simulink model "Refined_Model_1"  (R2020b)
settings: Solver=ode8  StartTime=0.0  StopTime=250  FixedStep=dt  RelTol=1e-3
values from neighbouring files (symbols this model uses):
  CovDist = RoadProfile(:,4)    [ICE_Val.m]
  Cx = VehicleDefine(7,3)    [BEV_Basictest.m]    (also in GPS_val.m; ICEBEV_Script.m; ICEBEV_Script_VECTO.m; ICE_Script.m)
  DynRolRad = VehicleDefine(5,3)    [BEV_Basictest.m]    (also in GPS_val.m; ICEBEV_Script.m; ICEBEV_Script_VECTO.m; ICE_Script.m)
  EngineRpm = round(IntpTorCur(:,1))    [GPS_val.m]    (also in ICEBEV_Script.m; ICEBEV_Script_VECTO.m; ICE_Script.m; ICE_Script_SSVal.m)
  etaClutch = VehicleDefine(23,3)    [GPS_val.m]    (also in ICEBEV_Script.m; ICEBEV_Script_VECTO.m; ICE_Script.m; ICE_Script_SSVal.m)
  etaGRa = GBXDefine(:,3)    [GPS_val.m]    (also in ICEBEV_Script.m; ICEBEV_Script_VECTO.m; ICE_Script.m; ICE_Script_SSVal.m)
  FDR = VehicleDefine(20,3)    [BEV_Basictest.m]    (also in GPS_val.m = VehicleDefine(22,3); ICEBEV_Script.m = VehicleDefine(22,3); ICEBEV_Script_VECTO.m = VehicleDefine(22,3); ICE_Script.m = VehicleDefine(22,3))
  Fr = VehicleDefine(13,3)    [BEV_Basictest.m]    (also in GPS_val.m; ICEBEV_Script.m; ICEBEV_Script_VECTO.m; ICE_Script.m)
  g = VehicleDefine(14,3)    [BEV_Basictest.m]    (also in GPS_val.m; ICEBEV_Script.m; ICEBEV_Script_VECTO.m; ICE_Script.m)
  GNo = GBXDefine(:,1)    [GPS_val.m]    (also in ICEBEV_Script.m; ICEBEV_Script_VECTO.m; ICE_Script.m; ICE_Script_SSVal.m)
  GRa = GBXDefine(:,2)    [GPS_val.m]    (also in ICEBEV_Script.m; ICEBEV_Script_VECTO.m; ICE_Script.m; ICE_Script_SSVal.m)
  InitVel = VehicleDefine(21,3)    [BEV_Basictest.m]    (also in GPS_val.m = VehicleDefine(24,3); ICEBEV_Script.m = VehicleDefine(24,3); ICEBEV_Script_VECTO.m = VehicleDefine(24,3); ICE_Script.m = VehicleDefine(24,3))
  IntpSlope = round(IntpSlope,1)    [GPS_val.m]    (also in ICE_Script.m; ICE_Val.m = A)
  Jk = VehicleDefine(15,3)    [BEV_Basictest.m]    (also in GPS_val.m; ICEBEV_Script.m; ICEBEV_Script_VECTO.m; ICE_Script.m)
  Jm = VehicleDefine(16,3)    [GPS_val.m]    (also in ICEBEV_Script.m; ICEBEV_Script_VECTO.m; ICE_Script.m; ICE_Script_SSVal.m)
  MaxSpeedProfile = FMSP    [GPS_val.m]    (also in ICE_Script.m; ICE_Val.m = repelem(SegSPLatinmps,SegLeninm))
  MaxTorValThrot = max(ThrotTableVal,[],2)    [GPS_val.m]    (also in ICEBEV_Script.m; ICEBEV_Script_VECTO.m; ICE_Script.m; ICE_Script_SSVal.m)
  Me = VehicleDefine(10,3)    [BEV_Basictest.m]    (also in GPS_val.m; ICEBEV_Script.m; ICEBEV_Script_VECTO.m; ICE_Script.m)
  MotoringTor = IntpTorCur(:,3)    [GPS_val.m]    (also in ICEBEV_Script.m; ICEBEV_Script_VECTO.m; ICE_Script.m; ICE_Script_SSVal.m)
  Mt = VehicleDefine(12,3)    [BEV_Basictest.m]    (also in GPS_val.m; ICEBEV_Script.m; ICEBEV_Script_VECTO.m; ICE_Script.m)
  Mtot = Mv+Me+Mt    [BEV_Basictest.m]    (also in GPS_val.m; ICEBEV_Script.m; ICEBEV_Script_VECTO.m; ICE_Script.m)
  Mv = VehicleDefine(9,3)    [BEV_Basictest.m]    (also in GPS_val.m; ICEBEV_Script.m; ICEBEV_Script_VECTO.m; ICE_Script.m)
  NoSteps = round(Dist(end))    [GPS_val.m]    (also in ICE_Script.m; ICE_Val.m = 3002)
  NoWhlFA = VehicleDefine(2,3)    [BEV_Basictest.m]    (also in GPS_val.m; ICE_Script.m; ICE_Val.m; ICE_Val_new.m)
  NoWhlRA = VehicleDefine(4,3)    [BEV_Basictest.m]    (also in GPS_val.m; ICE_Script.m; ICE_Val.m; ICE_Val_new.m)
  rho = VehicleDefine(6,3)    [BEV_Basictest.m]    (also in GPS_val.m; ICEBEV_Script.m; ICEBEV_Script_VECTO.m; ICE_Script.m)
  RpmBrkPnt = ThrottleMap(1,:)    [GPS_val.m]    (also in ICEBEV_Script.m; ICEBEV_Script_VECTO.m; ICE_Script.m; ICE_Script_SSVal.m)
  SegNo = RoadProfile(:,1)    [ICE_Val.m]
  SegSPLatinmps = (sqrt(aMaxLat*g*CurRadinm))    [GPS_val.m]    (also in ICE_Script.m; ICE_Val.m)
  Sx = VehicleDefine(8,3)    [BEV_Basictest.m]    (also in GPS_val.m; ICEBEV_Script.m; ICEBEV_Script_VECTO.m; ICE_Script.m)
  ThrotPos = ThrotPos'    [GPS_val.m]    (also in ICEBEV_Script.m; ICEBEV_Script_VECTO.m; ICE_Script.m; ICE_Script_SSVal.m)
  ThrotTableVal = ThrottleMap(2:end,2:end)    [GPS_val.m]    (also in ICEBEV_Script.m; ICEBEV_Script_VECTO.m; ICE_Script.m; ICE_Script_SSVal.m)
undefined symbols (not defined in the file or in its folder): AccLim, G1Inprpm, GearNo, GInprpm, GInpTor, GTorLoss, MaxSpinG, MaxWhlTorinG
libraries: simulink x2
settings Model: Creator=Kshitij  LastModifiedBy=Kshitij
settings SolverCC: AutoInsertRateTranBlk=on
settings DataIOCC: SaveFinalState=on  SaveState=on  InspectSignalLogs=on
settings DebuggingCC: AlgebraicLoopMsg=none
settings SFSimCC: SimTargetLang=C++  GPUAcceleration=on  SimDLTargetLibrary=cudnn

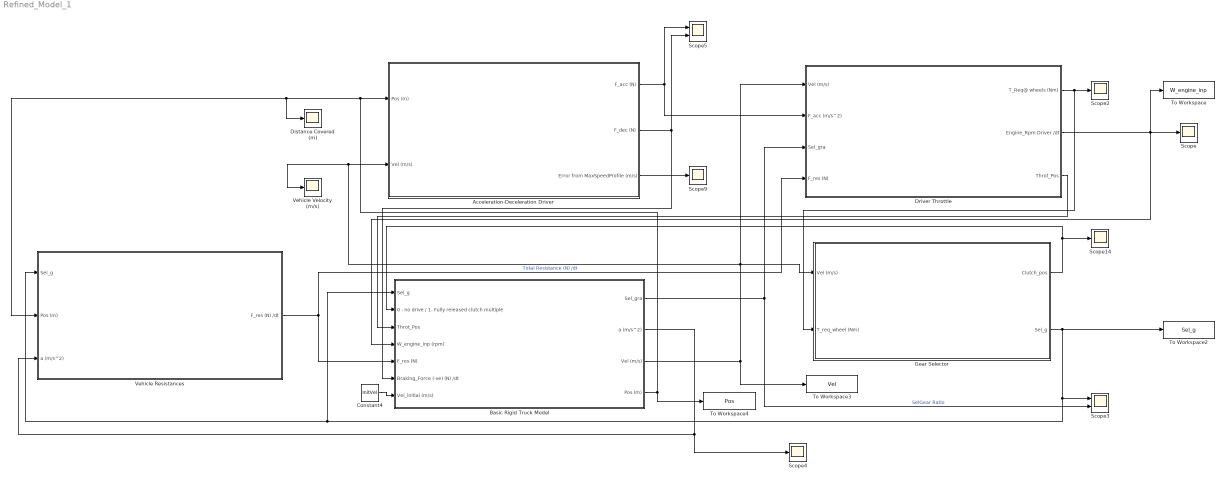
== system Refined_Model_1 ==
  Acceleration-Deceleration Driver : Subsystem
  Basic Rigid Truck Model : Subsystem
  Constant4 : Constant  Value=InitVel
  Distance Covered (m) : Scope
  Driver Throttle : Subsystem
  Gear Selector : Subsystem
  Scope{,2,4,9,14} (5 alike) : Scope
  Scope3 : Scope  NumInputPorts=2
  Scope5 : Scope  NumInputPorts=2
  To Workspace : ToWorkspace  VariableName=W_engine_inp  SaveFormat=Timeseries  SampleTime=-1
  To Workspace2 : ToWorkspace  VariableName=Sel_g  SaveFormat=Timeseries  SampleTime=-1
  To Workspace3 : ToWorkspace  VariableName=Vel  SaveFormat=Timeseries  SampleTime=-1
  To Workspace4 : ToWorkspace  VariableName=Pos  SaveFormat=Timeseries  SampleTime=-1
  Vehicle Resistances : Subsystem
  Vehicle Velocity (m/s) : Scope
  wires:
  Basic Rigid Truck Model/4(Pos (m)) -> Acceleration-Deceleration Driver/1(Pos (m)), Distance Covered (m)/1, Vehicle Resistances/2(Pos (m)), To Workspace4/1
  Vehicle Resistances/1(F_res (N) /dt) -> Basic Rigid Truck Model/5(F_res (N)), Driver Throttle/4(F_res (N))  "Total Resistance (N) /dt"
  Basic Rigid Truck Model/2(a (m/s^2)) -> Scope4/1, Vehicle Resistances/3(a (m/s^2))
  Gear Selector/1(Clutch_pos) -> Basic Rigid Truck Model/2(0 - no drive / 1- Fully released clutch multiple), Scope14/1
  Gear Selector/2(Sel_g) -> To Workspace2/1, Basic Rigid Truck Model/1(Sel_g), Vehicle Resistances/1(Sel_g), Scope3/1
  Acceleration-Deceleration Driver/3(Error from MaxSpeedProfile (m/s)) -> Scope9/1
  Acceleration-Deceleration Driver/2(F_dec (N)) -> Basic Rigid Truck Model/6(Braking_Force (-ve) (N) /dt), Scope5/2
  Basic Rigid Truck Model/1(Sel_gra) -> Driver Throttle/3(Sel_gra), Scope3/2  "SelGear Ratio"
  Acceleration-Deceleration Driver/1(F_acc (N)) -> Scope5/1, Driver Throttle/2(F_acc (m/s^2))
  Driver Throttle/2(Engine_Rpm Driver /dt) -> To Workspace/1, Scope/1, Basic Rigid Truck Model/4(W_engine_inp (rpm))
  Driver Throttle/1(T_Req@ wheels (Nm)) -> Gear Selector/2(T_req_wheel (Nm)), Scope2/1
  Constant4/1 -> Basic Rigid Truck Model/7(Vel_initial (m/s))
  Basic Rigid Truck Model/3(Vel (m/s)) -> Driver Throttle/1(Vel (m/s)), Vehicle Velocity (m/s)/1, Acceleration-Deceleration Driver/2(Vel (m/s)), Gear Selector/1(Vel (m/s)), To Workspace3/1
  Driver Throttle/3(Throt_Pos) -> Basic Rigid Truck Model/3(Throt_Pos)

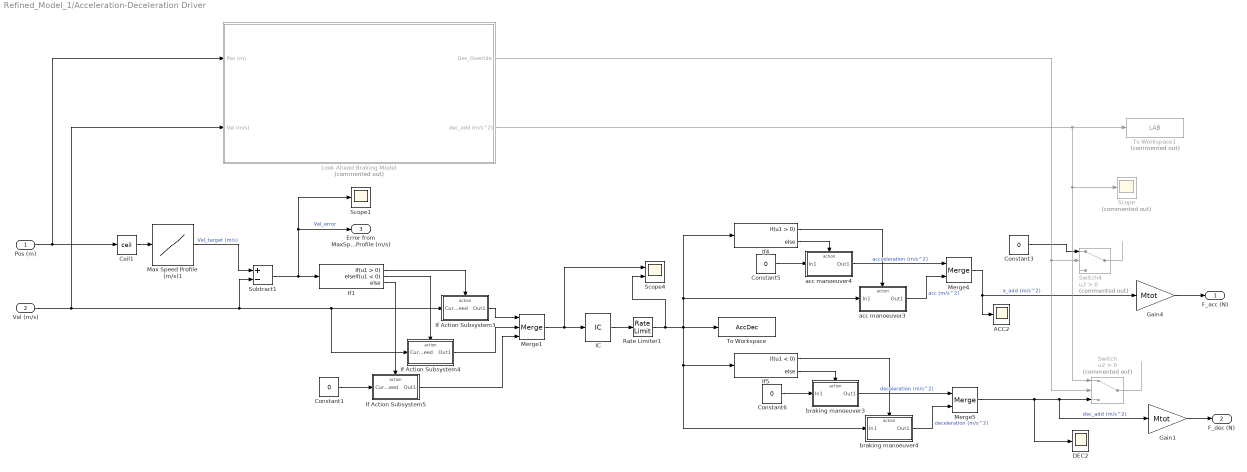
== system Refined_Model_1/Acceleration-Deceleration Driver ==
  Pos (m) : Inport
  Vel (m/s) : Inport  Port=2
  ACC2 : Scope
  Ceil1 : Rounding  Operator=ceil
  Constant{1,3,5..6} (4 alike) : Constant  Value=0
  DEC2 : Scope
  Gain1 : Gain  Gain=Mtot
  Gain4 : Gain  Gain=Mtot
  IC : InitialCondition  Value=0
  If Action Subsystem3 : Subsystem  TreatAsAtomicUnit=on
  If Action Subsystem4 : Subsystem  TreatAsAtomicUnit=on
  If Action Subsystem5 : Subsystem  TreatAsAtomicUnit=on
  If1 : If  ElseIfExpressions=u1 < 0
  If4 : If
  If5 : If  IfExpression=u1 < 0
  Look Ahead Braking Model : Subsystem  Commented=on
  Max Speed Profile (m/s)1 : Lookup_n-D  NumberOfTableDimensions=1  BreakpointsForDimension1=[1:length(MaxSpeedProfile)]  BreakpointsForDimension2=G1Inprpm  Table=MaxSpeedProfile  InterpMethod=Linear Lagrange  InternalRulePriority=Speed  RndMeth=Simplest  InputSameDT=on
  Merge1 : Merge  Inputs=3
  Merge4 : Merge
  Merge5 : Merge
  Rate Limiter1 : RateLimiter  RisingSlewLimit=0.5  SampleTimeMode=inherited
  Scope : Scope  Commented=on
  Scope1 : Scope
  Scope4 : Scope  NumInputPorts=2
  Subtract1 : Sum  Inputs=+-
  Switch : Switch  Commented=on  Criteria=u2 > Threshold
  Switch4 : Switch  Commented=on  Criteria=u2 > Threshold
  To Workspace : ToWorkspace  VariableName=AccDec  SaveFormat=Timeseries  SampleTime=-1
  To Workspace1 : ToWorkspace  Commented=on  VariableName=LAB  SaveFormat=Timeseries  SampleTime=-1
  acc manoeuver3 : Subsystem  TreatAsAtomicUnit=on
  acc manoeuver4 : Subsystem  TreatAsAtomicUnit=on
  braking manoeuver3 : Subsystem  TreatAsAtomicUnit=on
  braking manoeuver4 : Subsystem  TreatAsAtomicUnit=on
  F_acc (N) : Outport
  F_dec (N) : Outport  Port=2
  Error from MaxSpeedProfile (m/s) : Outport  Port=3
  wires:
  acc manoeuver4/1(Out1) -> Merge4/1  "accceleration (m/s^2)"
  If Action Subsystem3/1(Out1) -> Merge1/1
  If Action Subsystem5/1(Out1) -> Merge1/3
  Ceil1/1 -> Max Speed Profile (m/s)1/1
  If5/2 -> braking manoeuver3/Action
  Pos (m)/1 -> Look Ahead Braking Model/1(Pos (m)), Ceil1/1
  If1/1 -> If Action Subsystem3/Action
  If5/1 -> braking manoeuver4/Action
  Constant5/1 -> acc manoeuver4/1(In1)
  braking manoeuver3/1(Out1) -> Merge5/1  "deceleration (m/s^2)"
  braking manoeuver4/1(Out1) -> Merge5/2  "deceleration (m/s^2)"
  Constant6/1 -> braking manoeuver3/1(In1)
  Merge5/1 -> Gain1/1, Switch/3, DEC2/1  "dec_add (m/s^2)"
  If Action Subsystem4/1(Out1) -> Merge1/2
  acc manoeuver3/1(Out1) -> Merge4/2  "acc (m/s^2)"
  Merge4/1 -> ACC2/1, Gain4/1  "a_add (m/s^2)"
  If1/2 -> If Action Subsystem4/Action
  Subtract1/1 -> Error from MaxSpeedProfile (m/s)/1, Scope1/1, If1/1  "Vel_error"
  Rate Limiter1/1 -> Scope4/2, If4/1, acc manoeuver3/1(In1), If5/1, braking manoeuver4/1(In1), To Workspace/1
  If4/2 -> acc manoeuver4/Action
  If4/1 -> acc manoeuver3/Action
  If1/3 -> If Action Subsystem5/Action
  Merge1/1 -> IC/1, Scope4/1
  Max Speed Profile (m/s)1/1 -> Subtract1/1  "Vel_target (m/s)"
  Vel (m/s)/1 -> Look Ahead Braking Model/2(Vel (m/s)), If Action Subsystem4/1(Current Speed), If Action Subsystem3/1(Current Speed), Subtract1/2
  Constant1/1 -> If Action Subsystem5/1(Current Speed)
  IC/1 -> Rate Limiter1/1
  Constant3/1 -> Switch4/1
  Look Ahead Braking Model/1(Dec_Override) -> Switch/2, Switch4/2
  Look Ahead Braking Model/2(dec_add (m/s^2)) -> To Workspace1/1, Scope/1, Switch/1
  Gain4/1 -> F_acc (N)/1
  Switch4/1 -> ?
  Gain1/1 -> F_dec (N)/1
  Switch/1 -> ?

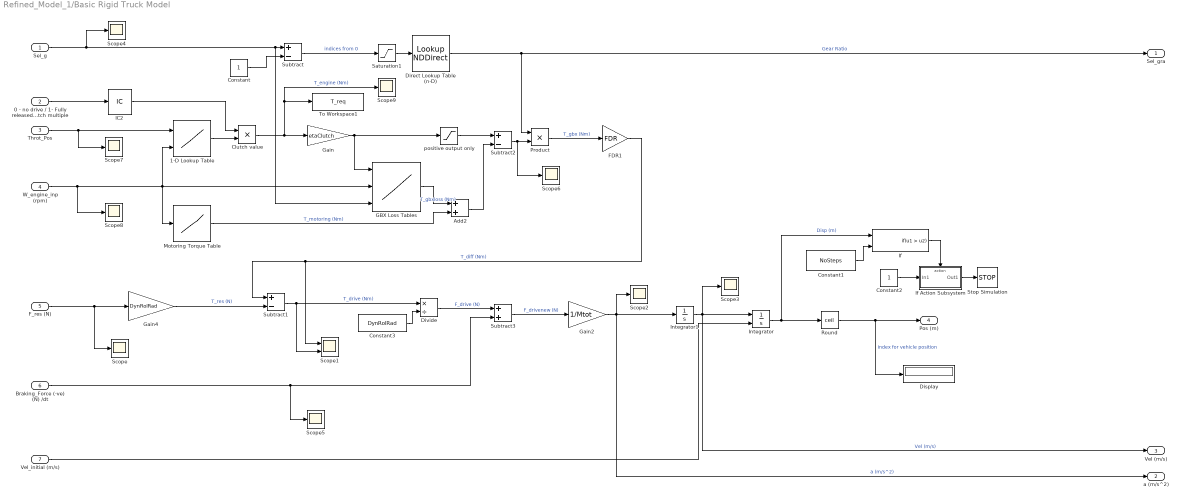
== system Refined_Model_1/Basic Rigid Truck Model ==
  Sel_g : Inport
  0 - no drive / 1- Fully released clutch multiple : Inport  Port=2
  Throt_Pos : Inport  Port=3
  W_engine_inp (rpm) : Inport  Port=4
  F_res (N) : Inport  Port=5
  Braking_Force (-ve) (N) /dt : Inport  Port=6
  Vel_initial (m/s) : Inport  Port=7
  1-D Lookup Table : Lookup_n-D  BreakpointsForDimension1=ThrotPos  BreakpointsForDimension2=RpmBrkPnt  Table=ThrotTableVal  InternalRulePriority=Speed  RndMeth=Simplest  InputSameDT=on
      settings: InputPortMap=u0,u1
  Add2 : Sum
  Clutch value : Product
  Constant : Constant
  Constant1 : Constant  Value=NoSteps
  Constant2 : Constant
  Constant3 : Constant  Value=DynRolRad
  Direct Lookup Table (n-D) : LookupNDDirect  NumberOfTableDimensions=1  Table=GRa
  Display : Display
  Divide : Product  Inputs=*/
  FDR1 : Gain  Gain=FDR
  GBX Loss Tables : Lookup_n-D  NumberOfTableDimensions=3  BreakpointsForDimension1=GInpTor  BreakpointsForDimension2=GInprpm  BreakpointsForDimension3=GearNo  Table=GTorLoss  InterpMethod=Linear Lagrange  InternalRulePriority=Speed  RndMeth=Simplest  InputSameDT=on
      settings: InputPortMap=u0,u1,u2
  Gain : Gain  Gain=etaClutch
  Gain2 : Gain  Gain=1/Mtot
  Gain4 : Gain  Gain=DynRolRad
  IC2 : InitialCondition
  If : If  NumInputs=2  IfExpression=u1 > u2  ShowElse=off
  If Action Subsystem : Subsystem  TreatAsAtomicUnit=on
  Integrator : Integrator  InitialConditionSource=external  ContinuousStateAttributes='velocity'
  Integrator1 : Integrator  ContinuousStateAttributes='acceleration'
  Motoring Torque Table : Lookup_n-D  NumberOfTableDimensions=1  BreakpointsForDimension1=EngineRpm  BreakpointsForDimension2=G1Inprpm  Table=MotoringTor  InterpMethod=Linear Lagrange  InternalRulePriority=Speed  RndMeth=Simplest  InputSameDT=on
  Product : Product
  Round : Rounding  Operator=ceil
  Saturation1 : Saturate  UpperLimit=inf  LowerLimit=0
  Scope{,2..9} (9 alike) : Scope
  Scope1 : Scope  NumInputPorts=2
  Stop Simulation : Stop
  Subtract : Sum  Inputs=+-
  Subtract1 : Sum  Inputs=+-
  Subtract2 : Sum  Inputs=+-
  Subtract3 : Sum
  To Workspace1 : ToWorkspace  VariableName=T_req  SaveFormat=Timeseries  SampleTime=-1
  positive output only : Saturate  UpperLimit=max(MaxTorValThrot)  LowerLimit=0
  Sel_gra : Outport
  a (m/s^2) : Outport  Port=2
  Vel (m/s) : Outport  Port=3
  Pos (m) : Outport  Port=4
  wires:
  GBX Loss Tables/1 -> Add2/1  "T_gbxloss (Nm)"
  Motoring Torque Table/1 -> Add2/2  "T_motoring (Nm)"
  FDR1/1 -> Subtract1/1, Scope1/1  "T_diff (Nm)"
  Direct Lookup Table (n-D)/1 -> Sel_gra/1, Product/1  "Gear Ratio"
  Clutch value/1 -> To Workspace1/1, Scope9/1, Gain/1  "T_engine (Nm)"
  Gain4/1 -> Subtract1/2  "T_res (N)"
  Subtract1/1 -> Divide/1, Scope1/2  "T_drive (Nm)"
  Add2/1 -> Subtract2/2
  Subtract2/1 -> Scope6/1, Product/2
  0 - no drive / 1- Fully released clutch multiple/1 -> IC2/1
  F_res (N)/1 -> Scope/1, Gain4/1
  Divide/1 -> Subtract3/1  "F_drive (N)"
  positive output only/1 -> Subtract2/1
  Sel_g/1 -> Scope4/1, Subtract/1, GBX Loss Tables/3
  Subtract/1 -> Saturation1/1  "indices from 0"
  Constant/1 -> Subtract/2
  Subtract3/1 -> Gain2/1  "F_drivenew (N)"
  Gain2/1 -> Integrator1/1, Scope2/1, a (m/s^2)/1  "a (m/s^2)"
  1-D Lookup Table/1 -> Clutch value/2
  Product/1 -> FDR1/1  "T_gbx (Nm)"
  Gain/1 -> positive output only/1, GBX Loss Tables/1
  W_engine_inp (rpm)/1 -> Scope8/1, Motoring Torque Table/1, GBX Loss Tables/2, 1-D Lookup Table/2
  IC2/1 -> Clutch value/1
  If/1 -> If Action Subsystem/Action
  Integrator1/1 -> Integrator/1, Scope3/1, Vel (m/s)/1  "Vel (m/s)"
  Constant1/1 -> If/2
  If Action Subsystem/1(Out1) -> Stop Simulation/1
  Round/1 -> Pos (m)/1, Display/1  "Index for vehicle position"
  Constant2/1 -> If Action Subsystem/1(In1)
  Integrator/1 -> Round/1, If/1  "Disp (m)"
  Constant3/1 -> Divide/2
  Vel_initial (m/s)/1 -> Integrator/2
  Saturation1/1 -> Direct Lookup Table (n-D)/1
  Throt_Pos/1 -> Scope7/1, 1-D Lookup Table/1
  Braking_Force (-ve) (N) /dt/1 -> Scope5/1, Subtract3/2

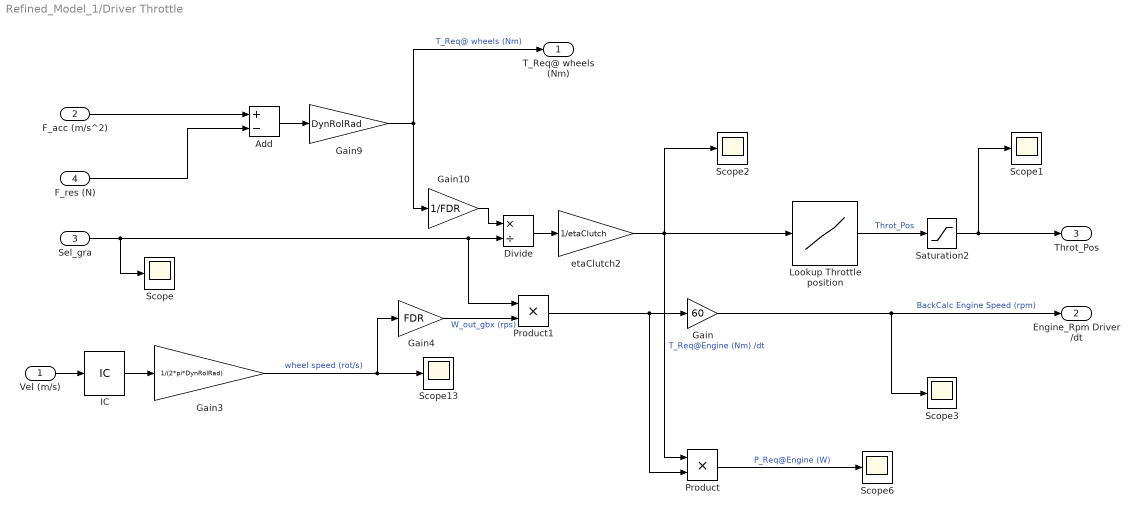
== system Refined_Model_1/Driver Throttle ==
  Vel (m/s) : Inport
  F_acc (m/s^2) : Inport  Port=2
  Sel_gra : Inport  Port=3
  F_res (N) : Inport  Port=4
  Add : Sum  Inputs=+-
  Divide : Product  Inputs=*/
  Gain : Gain  Gain=60
  Gain10 : Gain  Gain=1/FDR
  Gain3 : Gain  Gain=1/(2*pi*DynRolRad)
  Gain4 : Gain  Gain=FDR
  Gain9 : Gain  Gain=DynRolRad
  IC : InitialCondition  Value=0.1
  Lookup Throttle position : Lookup_n-D  NumberOfTableDimensions=1  BreakpointsForDimension1=MaxTorValThrot  Table=ThrotPos  InternalRulePriority=Speed  RndMeth=Simplest  InputSameDT=on
  Product : Product
  Product1 : Product
  Saturation2 : Saturate  UpperLimit=1  LowerLimit=0
  Scope{,1..3,6,13} (6 alike) : Scope
  etaClutch2 : Gain  Gain=1/etaClutch
  T_Req@ wheels (Nm) : Outport
  Engine_Rpm Driver /dt : Outport  Port=2
  Throt_Pos : Outport  Port=3
  wires:
  etaClutch2/1 -> Scope2/1, Lookup Throttle position/1, Product/1  "T_Req@Engine (Nm) /dt"
  Add/1 -> Gain9/1
  Gain4/1 -> Product1/2  "W_out_gbx (rps)"
  Product/1 -> Scope6/1  "P_Req@Engine (W)"
  Gain9/1 -> Gain10/1, T_Req@ wheels (Nm)/1  "T_Req@ wheels (Nm)"
  Gain3/1 -> Scope13/1, Gain4/1  "wheel speed (rot/s)"
  Gain10/1 -> Divide/1
  Sel_gra/1 -> Scope/1, Divide/2, Product1/1
  F_acc (m/s^2)/1 -> Add/1
  Vel (m/s)/1 -> IC/1
  Divide/1 -> etaClutch2/1
  F_res (N)/1 -> Add/2
  Product1/1 -> Gain/1, Product/2
  Lookup Throttle position/1 -> Saturation2/1  "Throt_Pos"
  Saturation2/1 -> Scope1/1, Throt_Pos/1
  IC/1 -> Gain3/1
  Gain/1 -> Engine_Rpm Driver /dt/1, Scope3/1  "BackCalc Engine Speed (rpm)"

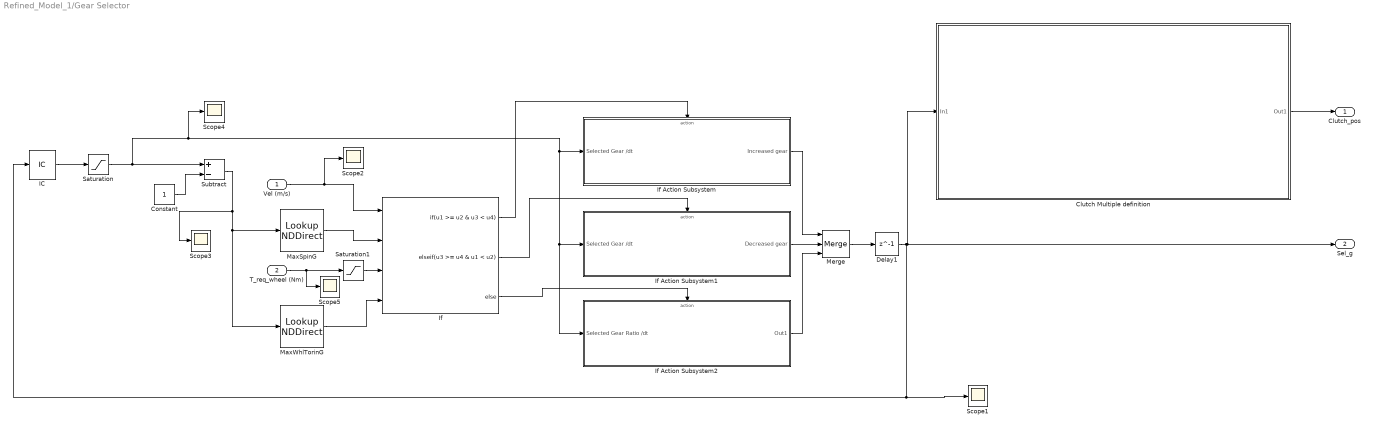
== system Refined_Model_1/Gear Selector ==
  Vel (m/s) : Inport
  T_req_wheel (Nm) : Inport  Port=2
  Clutch Multiple definition : Subsystem
  Constant : Constant
  Delay1 : Delay  DelayLength=1
  IC : InitialCondition
  If : If  NumInputs=4  IfExpression=u1 >= u2 & u3 < u4  ElseIfExpressions=u3 >= u4 & u1 < u2
  If Action Subsystem : Subsystem  TreatAsAtomicUnit=on
  If Action Subsystem1 : Subsystem  TreatAsAtomicUnit=on
  If Action Subsystem2 : Subsystem  TreatAsAtomicUnit=on
  MaxSpinG : LookupNDDirect  NumberOfTableDimensions=1  Table=MaxSpinG
  MaxWhlTorinG : LookupNDDirect  NumberOfTableDimensions=1  Table=MaxWhlTorinG
  Merge : Merge  Inputs=3
  Saturation : Saturate  UpperLimit=max(GNo)  LowerLimit=0
  Saturation1 : Saturate  UpperLimit=inf  LowerLimit=0
  Scope{1..5} (5 alike) : Scope
  Subtract : Sum  Inputs=+-
  Clutch_pos : Outport
  Sel_g : Outport  Port=2
  wires:
  If/1 -> If Action Subsystem/Action
  MaxWhlTorinG/1 -> If/4
  Vel (m/s)/1 -> Scope2/1, If/1
  MaxSpinG/1 -> If/2
  If/2 -> If Action Subsystem1/Action
  If Action Subsystem/1(Increased gear) -> Merge/1
  If Action Subsystem1/1(Decreased gear) -> Merge/2
  Constant/1 -> Subtract/2
  Subtract/1 -> Scope3/1, MaxSpinG/1, MaxWhlTorinG/1
  If/3 -> If Action Subsystem2/Action
  If Action Subsystem2/1(Out1) -> Merge/3
  Delay1/1 -> Clutch Multiple definition/1(In1), Sel_g/1, IC/1, Scope1/1
  Saturation/1 -> Subtract/1, If Action Subsystem2/1(Selected Gear Ratio /dt), If Action Subsystem1/1(Selected Gear /dt), If Action Subsystem/1(Selected Gear /dt), Scope4/1
  T_req_wheel (Nm)/1 -> Scope5/1, Saturation1/1
  Clutch Multiple definition/1(Out1) -> Clutch_pos/1
  Saturation1/1 -> If/3
  Merge/1 -> Delay1/1
  IC/1 -> Saturation/1

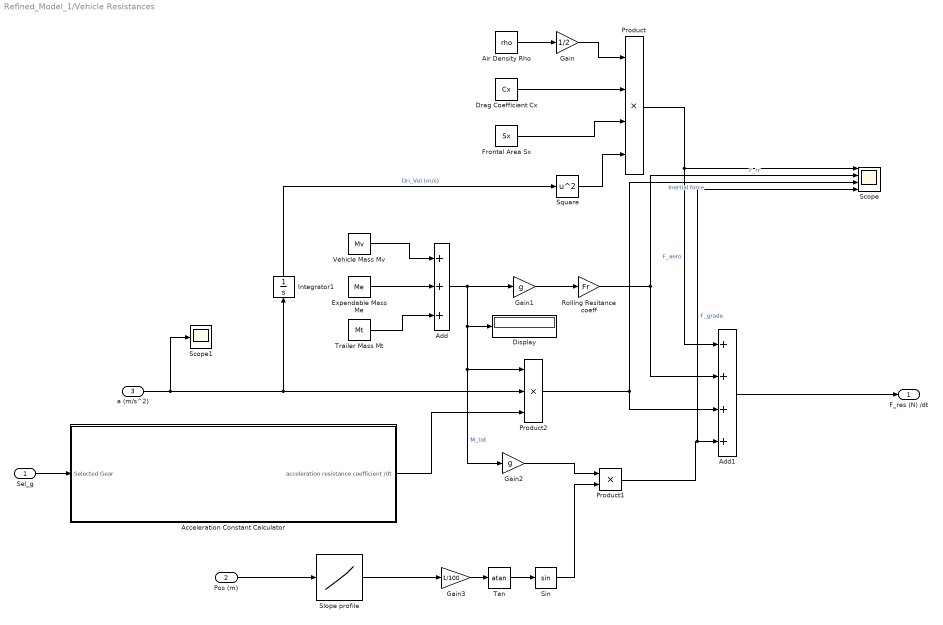
== system Refined_Model_1/Vehicle Resistances ==
  Sel_g : Inport
  Pos (m) : Inport  Port=2
  a (m/s^2) : Inport  Port=3
  Acceleration Constant Calculator : Subsystem
  Add : Sum  Inputs=+++
  Add1 : Sum  Inputs=++++
  Air Density Rho : Constant  Value=rho
  Display : Display
  Drag Coefficient Cx : Constant  Value=Cx
  Expendable Mass Me : Constant  Value=Me
  Frontal Area Sx : Constant  Value=Sx
  Gain : Gain  Gain=1/2
  Gain1 : Gain  Gain=g
  Gain2 : Gain  Gain=g
  Gain3 : Gain  Gain=1/100
  Integrator1 : Integrator
  Product : Product  Inputs=4
  Product1 : Product
  Product2 : Product  Inputs=3
  Rolling Resitance coeff : Gain  Gain=Fr
  Scope : Scope  NumInputPorts=4
  Scope1 : Scope
  Sin : Trigonometry
  Slope profile : Lookup_n-D  NumberOfTableDimensions=1  BreakpointsForDimension1=1: length(IntpSlope)  Table=IntpSlope  InternalRulePriority=Speed  RndMeth=Simplest  InputSameDT=on
  Square : Math  Operator=square  SaturateOnIntegerOverflow=on
  Tan : Trigonometry  Operator=atan
  Trailer Mass Mt : Constant  Value=Mt
  Vehicle Mass Mv : Constant  Value=Mv
  F_res (N) /dt : Outport
  wires:
  Expendable Mass Me/1 -> Add/2
  Add/1 -> Display/1, Gain2/1, Product2/1, Gain1/1  "M_tot"
  Gain/1 -> Product/1
  Sin/1 -> Product1/2
  Tan/1 -> Sin/1
  Product1/1 -> Scope/4, Add1/4  "F_grade"
  Air Density Rho/1 -> Gain/1
  Drag Coefficient Cx/1 -> Product/2
  Integrator1/1 -> Square/1  "Dri_Vel (m/s)"
  Pos (m)/1 -> Slope profile/1
  Gain2/1 -> Product1/1
  Trailer Mass Mt/1 -> Add/3
  Rolling Resitance coeff/1 -> Scope/2, Add1/2  "F_rr"
  Square/1 -> Product/4
  Gain1/1 -> Rolling Resitance coeff/1
  Vehicle Mass Mv/1 -> Add/1
  Product/1 -> Scope/1, Add1/1  "F_aero"
  Gain3/1 -> Tan/1
  Frontal Area Sx/1 -> Product/3
  Product2/1 -> Scope/3, Add1/3  "Inertial force"
  Acceleration Constant Calculator/1(acceleration resistance coefficient /dt) -> Product2/3
  Sel_g/1 -> Acceleration Constant Calculator/1(Selected Gear)
  Add1/1 -> F_res (N) /dt/1
  a (m/s^2)/1 -> Scope1/1, Product2/2, Integrator1/1
  Slope profile/1 -> Gain3/1

== system Refined_Model_1/Acceleration-Deceleration Driver/If Action Subsystem3 ==
  Current Speed : Inport
  Action Port : ActionPort  ActionPortLabel=if(u1 > 0)
  Acceleration : Lookup_n-D  NumberOfTableDimensions=1  BreakpointsForDimension1=AccLim(:,1)  Table=AccLim(:,2)  InternalRulePriority=Speed  RndMeth=Simplest  InputSameDT=on
  Out1 : Outport
  wires:
  Current Speed/1 -> Acceleration/1
  Acceleration/1 -> Out1/1  "Acceleration in m/s^2"

== system Refined_Model_1/Acceleration-Deceleration Driver/If Action Subsystem4 ==
  Current Speed : Inport
  Action Port : ActionPort  ActionPortLabel=elseif(u1 < 0)
  Deceleration : Lookup_n-D  NumberOfTableDimensions=1  BreakpointsForDimension1=AccLim(:,1)  Table=AccLim(:,3)  InternalRulePriority=Speed  RndMeth=Simplest  InputSameDT=on
  Out1 : Outport
  wires:
  Deceleration/1 -> Out1/1  "Acceleration in m/s^2"
  Current Speed/1 -> Deceleration/1

== system Refined_Model_1/Acceleration-Deceleration Driver/If Action Subsystem5 ==
  Current Speed : Inport
  Action Port : ActionPort  ActionPortLabel=else
  Out1 : Outport
  wires:
  Current Speed/1 -> Out1/1  "Acceleration in m/s^2"

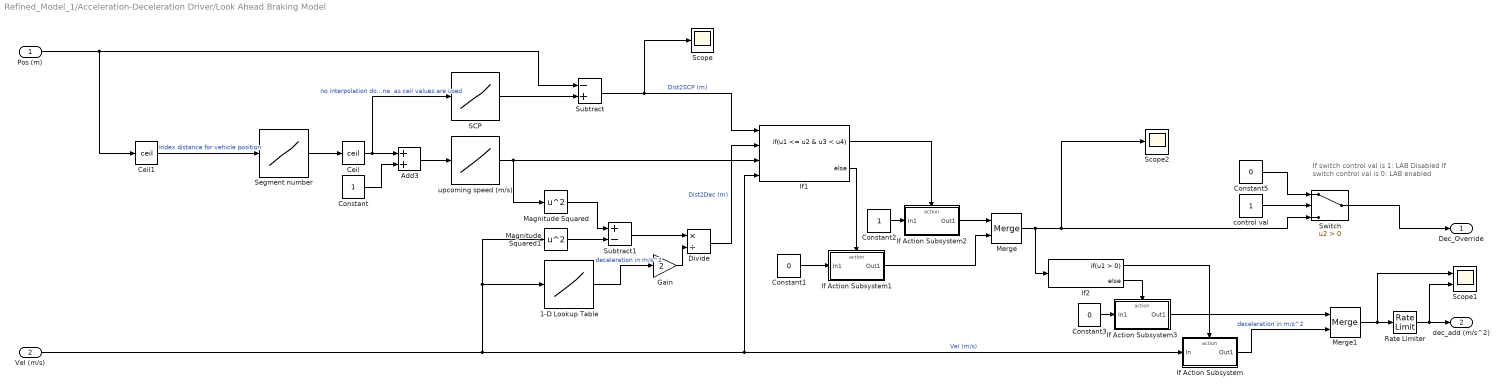
== system Refined_Model_1/Acceleration-Deceleration Driver/Look Ahead Braking Model ==
  note: If switch control val is 1: LAB Disabled
      | If switch control val is 0: LAB enabled
  Pos (m) : Inport
  Vel (m/s) : Inport  Port=2
  1-D Lookup Table : Lookup_n-D  NumberOfTableDimensions=1  BreakpointsForDimension1=AccLim(:,1)  Table=AccLim(:,3)  InternalRulePriority=Speed  RndMeth=Simplest  InputSameDT=on
  Add3 : Sum
  Ceil : Rounding  Operator=ceil
  Ceil1 : Rounding  Operator=ceil
  Constant : Constant
  Constant1 : Constant  Value=0
  Constant2 : Constant
  Constant3 : Constant  Value=0
  Constant5 : Constant  Value=0
  Divide : Product  Inputs=*/
  Gain : Gain  Gain=2
  If Action Subsystem : Subsystem  TreatAsAtomicUnit=on
  If Action Subsystem1 : Subsystem  TreatAsAtomicUnit=on
  If Action Subsystem2 : Subsystem  TreatAsAtomicUnit=on
  If Action Subsystem3 : Subsystem  TreatAsAtomicUnit=on
  If1 : If  NumInputs=4  IfExpression=u1 <= u2 & u3 < u4
  If2 : If
  Magnitude Squared : Math  Operator=square  SaturateOnIntegerOverflow=on
  Magnitude Squared1 : Math  Operator=square  SaturateOnIntegerOverflow=on
  Merge : Merge
  Merge1 : Merge
  Rate Limiter : RateLimiter  SampleTimeMode=inherited
  SCP : Lookup_n-D  NumberOfTableDimensions=1  BreakpointsForDimension1=SegNo  BreakpointsForDimension2=G1Inprpm  Table=CovDist  InterpMethod=Linear Lagrange  InternalRulePriority=Speed  RndMeth=Simplest  InputSameDT=on
  Scope : Scope
  Scope1 : Scope  NumInputPorts=2
  Scope2 : Scope
  Segment number : Lookup_n-D  NumberOfTableDimensions=1  BreakpointsForDimension1=CovDist  BreakpointsForDimension2=G1Inprpm  Table=SegNo  InterpMethod=Linear Lagrange  InternalRulePriority=Speed  RndMeth=Simplest  InputSameDT=on
  Subtract : Sum  Inputs=-+
  Subtract1 : Sum  Inputs=+-
  Switch : Switch  Criteria=u2 > Threshold
  control val : Constant
  upcoming speed (m/s) : Lookup_n-D  NumberOfTableDimensions=1  BreakpointsForDimension1=SegNo  BreakpointsForDimension2=G1Inprpm  Table=SegSPLatinmps  InterpMethod=Linear Lagrange  InternalRulePriority=Speed  RndMeth=Simplest  InputSameDT=on
  Dec_Override : Outport
  dec_add (m/s^2) : Outport  Port=2
  wires:
  Add3/1 -> upcoming speed (m/s)/1
  Ceil/1 -> SCP/1, Add3/1  "no interpolation done  as ceil values are used"
  SCP/1 -> Subtract/2
  upcoming speed (m/s)/1 -> If1/3, Magnitude Squared/1
  Constant/1 -> Add3/2
  Subtract/1 -> Scope/1, If1/1  "Dist2SCP (m)"
  Segment number/1 -> Ceil/1
  Ceil1/1 -> Segment number/1  "Index distance for vehicle position"
  Magnitude Squared/1 -> Subtract1/1
  Subtract1/1 -> Divide/1
  Gain/1 -> Divide/2
  1-D Lookup Table/1 -> Gain/1  "deceleration in m/s^2"
  Divide/1 -> If1/2  "Dist2Dec (m)"
  Vel (m/s)/1 -> 1-D Lookup Table/1, Magnitude Squared1/1, If Action Subsystem/1(In), If1/4  "Vel (m/s)"
  If Action Subsystem/1(Out1) -> Merge1/2  "deceleration in m/s^2"
  If1/2 -> If Action Subsystem1/Action
  Constant1/1 -> If Action Subsystem1/1(In1)
  Constant2/1 -> If Action Subsystem2/1(In1)
  If1/1 -> If Action Subsystem2/Action
  If Action Subsystem2/1(Out1) -> Merge/1
  If Action Subsystem1/1(Out1) -> Merge/2
  Merge/1 -> If2/1, Switch/3, Scope2/1
  If2/1 -> If Action Subsystem/Action
  If2/2 -> If Action Subsystem3/Action
  Constant3/1 -> If Action Subsystem3/1(In1)
  If Action Subsystem3/1(Out1) -> Merge1/1
  Magnitude Squared1/1 -> Subtract1/2
  Pos (m)/1 -> Ceil1/1, Subtract/1
  Merge1/1 -> Rate Limiter/1, Scope1/1
  Rate Limiter/1 -> Scope1/2, dec_add (m/s^2)/1
  control val/1 -> Switch/2
  Switch/1 -> Dec_Override/1
  Constant5/1 -> Switch/1

== system Refined_Model_1/Acceleration-Deceleration Driver/acc manoeuver3 ==
  In1 : Inport
  Action Port : ActionPort  ActionPortLabel=if(u1 > 0)
  Out1 : Outport
  wires:
  In1/1 -> Out1/1

== system Refined_Model_1/Acceleration-Deceleration Driver/acc manoeuver4 ==
  In1 : Inport
  Action Port : ActionPort  ActionPortLabel=else
  Out1 : Outport
  wires:
  In1/1 -> Out1/1

== system Refined_Model_1/Acceleration-Deceleration Driver/braking manoeuver3 ==
  In1 : Inport
  Action Port : ActionPort  ActionPortLabel=else
  Out1 : Outport
  wires:
  In1/1 -> Out1/1

== system Refined_Model_1/Acceleration-Deceleration Driver/braking manoeuver4 ==
  In1 : Inport
  Action Port : ActionPort  ActionPortLabel=if(u1 < 0)
  Out1 : Outport
  wires:
  In1/1 -> Out1/1

== system Refined_Model_1/Basic Rigid Truck Model/If Action Subsystem ==
  In1 : Inport
  Action Port : ActionPort  ActionPortLabel=if(u1 > u2)
  Out1 : Outport
  wires:
  In1/1 -> Out1/1

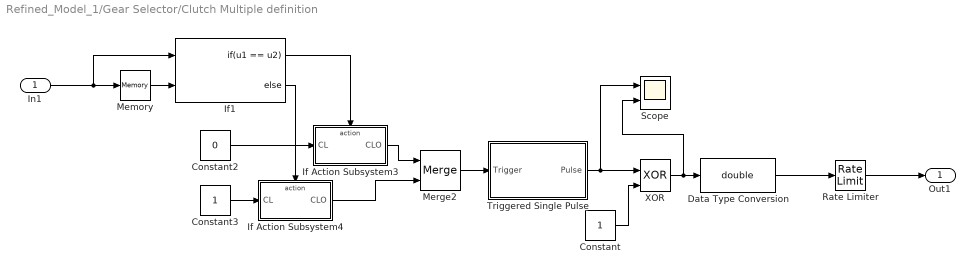
== system Refined_Model_1/Gear Selector/Clutch Multiple definition ==
  In1 : Inport
  Constant : Constant
  Constant2 : Constant  Value=0
  Constant3 : Constant
  Data Type Conversion : DataTypeConversion  OutDataTypeStr=double
  If Action Subsystem3 : Subsystem  TreatAsAtomicUnit=on
  If Action Subsystem4 : Subsystem  TreatAsAtomicUnit=on
  If1 : If  NumInputs=2  IfExpression=u1 == u2
  Memory : Memory
  Merge2 : Merge
  Rate Limiter : RateLimiter  SampleTimeMode=inherited
  Scope : Scope  NumInputPorts=2
  Triggered Single Pulse : Subsystem  TreatAsAtomicUnit=on  mask(single pulse generation){p_wid=10}
      mask prompts: p_wid "pulse width (number of samples)"
      mask help: This block generate a single pulse whenever a trigger happen. The pulse width must specified as a number of samples. for example if your sampling time is 0.1s and you want 3s pulse , then you should enter 30 as a pulse width.
      mask Display:
      | plot([0],[0])
      | plot([11],[0])
      | plot([5],[0.5])
      | plot([4 5 5 6 6 7],[0 0 0.25 0.25 0 0])
      | plot([5],[-0.3])
      | 
      | port_label('output', 1, 'Pulse')
      | port_label('input', 1, 'Trigger')
  XOR : Logic  Operator=XOR  IconShape=distinctive  AllPortsSameDT=off  OutDataTypeStr=boolean
  Out1 : Outport
  wires:
  If1/1 -> If Action Subsystem3/Action
  If Action Subsystem3/1(CLO) -> Merge2/1
  Memory/1 -> If1/2
  Constant2/1 -> If Action Subsystem3/1(CL)
  Constant3/1 -> If Action Subsystem4/1(CL)
  In1/1 -> Memory/1, If1/1
  If1/2 -> If Action Subsystem4/Action
  If Action Subsystem4/1(CLO) -> Merge2/2
  Merge2/1 -> Triggered Single Pulse/1(Trigger)
  Triggered Single Pulse/1(Pulse) -> Scope/1, XOR/1
  Rate Limiter/1 -> Out1/1
  Constant/1 -> XOR/2
  XOR/1 -> Scope/2, Data Type Conversion/1
  Data Type Conversion/1 -> Rate Limiter/1

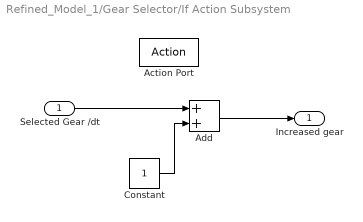
== system Refined_Model_1/Gear Selector/If Action Subsystem ==
  Selected Gear /dt : Inport
  Action Port : ActionPort  ActionPortLabel=if(u1 >= u2 & u3 < u4)
  Add : Sum
  Constant : Constant
  Increased gear : Outport
  wires:
  Selected Gear /dt/1 -> Add/1
  Add/1 -> Increased gear/1
  Constant/1 -> Add/2

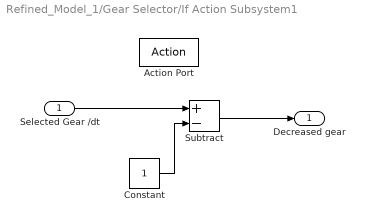
== system Refined_Model_1/Gear Selector/If Action Subsystem1 ==
  Selected Gear /dt : Inport
  Action Port : ActionPort  ActionPortLabel=elseif(u3 >= u4 & u1 < u2)
  Constant : Constant
  Subtract : Sum  Inputs=+-
  Decreased gear : Outport
  wires:
  Constant/1 -> Subtract/2
  Subtract/1 -> Decreased gear/1
  Selected Gear /dt/1 -> Subtract/1

== system Refined_Model_1/Gear Selector/If Action Subsystem2 ==
  Selected Gear Ratio /dt : Inport
  Action Port : ActionPort  ActionPortLabel=else
  Out1 : Outport
  wires:
  Selected Gear Ratio /dt/1 -> Out1/1

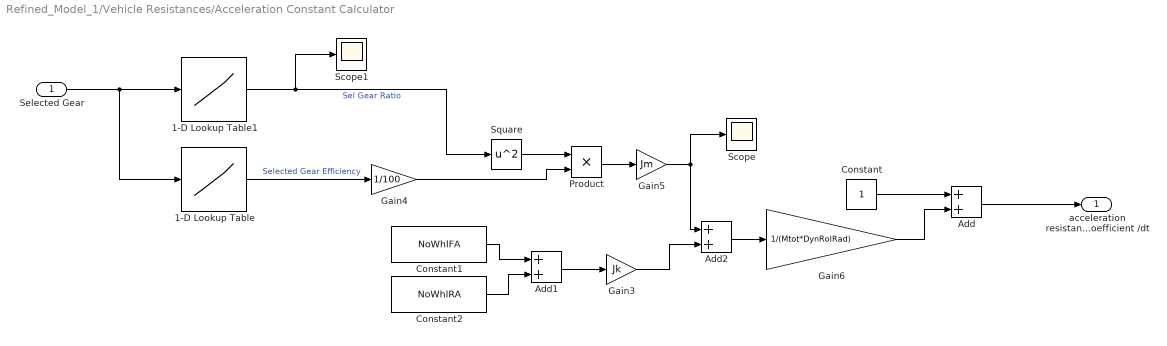
== system Refined_Model_1/Vehicle Resistances/Acceleration Constant Calculator ==
  Selected Gear : Inport
  1-D Lookup Table : Lookup_n-D  NumberOfTableDimensions=1  BreakpointsForDimension1=GNo  Table=etaGRa  InternalRulePriority=Speed  RndMeth=Simplest  InputSameDT=on
  1-D Lookup Table1 : Lookup_n-D  NumberOfTableDimensions=1  BreakpointsForDimension1=GNo  Table=GRa  InternalRulePriority=Speed  RndMeth=Simplest  InputSameDT=on
  Add : Sum
  Add1 : Sum
  Add2 : Sum
  Constant : Constant
  Constant1 : Constant  Value=NoWhlFA
  Constant2 : Constant  Value=NoWhlRA
  Gain3 : Gain  Gain=Jk
  Gain4 : Gain  Gain=1/100
  Gain5 : Gain  Gain=Jm
  Gain6 : Gain  Gain=1/(Mtot*DynRolRad)
  Product : Product
  Scope : Scope
  Scope1 : Scope
  Square : Math  Operator=square  SaturateOnIntegerOverflow=on
  acceleration resistance coefficient /dt : Outport
  wires:
  1-D Lookup Table/1 -> Gain4/1  "Selected Gear Efficiency"
  Add1/1 -> Gain3/1
  Product/1 -> Gain5/1
  Gain6/1 -> Add/2
  Square/1 -> Product/1
  Constant2/1 -> Add1/2
  Constant/1 -> Add/1
  Gain3/1 -> Add2/2
  Add2/1 -> Gain6/1
  Constant1/1 -> Add1/1
  Gain4/1 -> Product/2
  Gain5/1 -> Add2/1, Scope/1
  Selected Gear/1 -> 1-D Lookup Table/1, 1-D Lookup Table1/1
  1-D Lookup Table1/1 -> Scope1/1, Square/1  "Sel Gear Ratio"
  Add/1 -> acceleration resistance coefficient /dt/1

== system Refined_Model_1/Acceleration-Deceleration Driver/Look Ahead Braking Model/If Action Subsystem ==
  In : Inport
  Action Port : ActionPort  ActionPortLabel=if(u1 > 0)
  1-D Lookup Table : Lookup_n-D  NumberOfTableDimensions=1  BreakpointsForDimension1=AccLim(:,1)  Table=AccLim(:,3)  InternalRulePriority=Speed  RndMeth=Simplest  InputSameDT=on
  Out1 : Outport
  wires:
  In/1 -> 1-D Lookup Table/1
  1-D Lookup Table/1 -> Out1/1  "deceleration in m/s^2"

== system Refined_Model_1/Acceleration-Deceleration Driver/Look Ahead Braking Model/If Action Subsystem1 ==
  In1 : Inport
  Action Port : ActionPort  ActionPortLabel=else
  Out1 : Outport
  wires:
  In1/1 -> Out1/1

== system Refined_Model_1/Acceleration-Deceleration Driver/Look Ahead Braking Model/If Action Subsystem2 ==
  In1 : Inport
  Action Port : ActionPort  ActionPortLabel=if(u1 <= u2 & u3 < u4)
  Out1 : Outport
  wires:
  In1/1 -> Out1/1

== system Refined_Model_1/Acceleration-Deceleration Driver/Look Ahead Braking Model/If Action Subsystem3 ==
  In1 : Inport
  Action Port : ActionPort  ActionPortLabel=else
  Out1 : Outport
  wires:
  In1/1 -> Out1/1

== system Refined_Model_1/Gear Selector/Clutch Multiple definition/If Action Subsystem3 ==
  CL : Inport
  Action Port : ActionPort  ActionPortLabel=if(u1 == u2)
  CLO : Outport
  wires:
  CL/1 -> CLO/1

== system Refined_Model_1/Gear Selector/Clutch Multiple definition/If Action Subsystem4 ==
  CL : Inport
  Action Port : ActionPort  ActionPortLabel=else
  CLO : Outport
  wires:
  CL/1 -> CLO/1

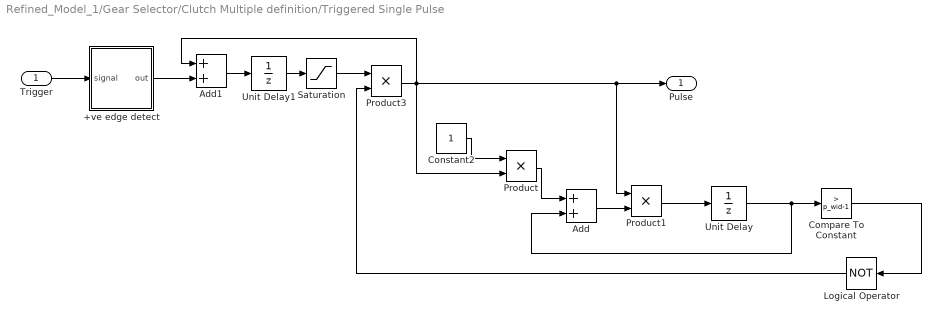
== system Refined_Model_1/Gear Selector/Clutch Multiple definition/Triggered Single Pulse ==
  Trigger : Inport
  +ve edge detect : Subsystem
  Add : Sum
  Add1 : Sum
  Compare To Constant : simulink/Logic and Bit Operations/Compare To Constant  relop=>  const=p_wid-1  OutDataTypeStr=boolean
  Constant2 : Constant
  Logical Operator : Logic  Operator=NOT  AllPortsSameDT=off  OutDataTypeStr=boolean
  Product : Product  RndMeth=Zero
  Product1 : Product  RndMeth=Zero
  Product3 : Product  RndMeth=Zero
  Saturation : Saturate  UpperLimit=1  LowerLimit=0
  Unit Delay : UnitDelay  SampleTime=-1  HasFrameUpgradeWarning=on
  Unit Delay1 : UnitDelay  SampleTime=-1  HasFrameUpgradeWarning=on
  Pulse : Outport
  wires:
  Compare To Constant/1 -> Logical Operator/1
  Constant2/1 -> Product/1
  Product/1 -> Add/1
  Unit Delay/1 -> Add/2, Compare To Constant/1
  Trigger/1 -> +ve edge detect/1(signal)
  +ve edge detect/1(out) -> Add1/2
  Add/1 -> Product1/2
  Product1/1 -> Unit Delay/1
  Add1/1 -> Unit Delay1/1
  Unit Delay1/1 -> Saturation/1
  Saturation/1 -> Product3/1
  Product3/1 -> Add1/1, Product/2, Product1/1, Pulse/1
  Logical Operator/1 -> Product3/2

== system Refined_Model_1/Gear Selector/Clutch Multiple definition/Triggered Single Pulse/+ve edge detect ==
  note: Edge
  signal : Inport
  Delay Input1 : UnitDelay  Description=Store in Global RAM  DisableCoverage=on  SampleTime=-1  HasFrameUpgradeWarning=on
  FixPt Relational Operator : RelationalOperator  Operator=>  OutDataTypeStr=fixdt(0, 8)  ZeroCross=off  RndMeth=Nearest
  Positive : simulink/Logic and Bit Operations/Compare To Zero  relop=>  OutDataTypeStr=uint8  ZeroCross=off
  out : Outport
  wires:
  Delay Input1/1 -> FixPt Relational Operator/2  "U(k-1)"
  Positive/1 -> Delay Input1/1, FixPt Relational Operator/1  "U(k)"
  FixPt Relational Operator/1 -> out/1
  signal/1 -> Positive/1
